simulink model "simTwoLinkFDIbasisComparison"  (R2014b)
settings: Solver=ode45  StartTime=0.0  StopTime=tof  FixedStep=dt  MaxStep=dtmax  RelTol=1e-3
values from neighbouring files (symbols this model uses):
  As = zeros(nofstates,nofstates)    [threeLinkFTC.m]    (also in twoLinkFDIbasisComparison.m; twoLinkFTC.m; twoLinkFTCwAdaptive.m)
  c1 = 0    [robotArmWith2Links.m]    (also in twoLinkFDIbasisComparison.m = 1; twoLinkFTC.m; twoLinkFTCwAdaptive.m)
  c2 = 0    [robotArmWith2Links.m]    (also in twoLinkFDIbasisComparison.m = 1; twoLinkFTC.m; twoLinkFTCwAdaptive.m)
  Dhat0 = zeros(6,1)    [threeLinkFTC.m]    (also in twoLinkFDIbasisComparison.m = zeros(4,1); twoLinkFTC.m = zeros(4,1); twoLinkFTCwAdaptive.m = zeros(4,1))
  dtFc = 1*dtmax    (= 0.001)    [threeLinkFTC.m]    (also in twoLinkFDIbasisComparison.m; twoLinkFTC.m; twoLinkFTCwAdaptive.m)
  epsilontheta = 0.01    [threeLinkFTC.m]    (also in twoLinkFDIbasisComparison.m; twoLinkFTC.m; twoLinkFTCwAdaptive.m)
  fault_gamma = 1    [twoLinkFDIbasisComparison.m]
  fault_taumax = 15    [twoLinkFDIbasisComparison.m]
  faultyArm = 3    [threeLinkFTC.m]    (also in twoLinkFDIbasisComparison.m = 2; twoLinkFTC.m = 2; twoLinkFTCwAdaptive.m = 1)
  g = 9.81    [robotArmWith2Links.m]    (also in threeLinkFTC.m; twoLinkFDIbasisComparison.m; twoLinkFTC.m; twoLinkFTCwAdaptive.m)
  GammaW = 1000    [threeLinkFTC.m]    (also in twoLinkFDIbasisComparison.m; twoLinkFTC.m; twoLinkFTCwAdaptive.m)
  I1 = 8.33e-2    (= 0.0833)    [robotArmWith2Links.m]    (also in threeLinkFTC.m = 0.0833333333333; twoLinkFDIbasisComparison.m = 0.0833333333333; twoLinkFTC.m = 0.0833333333333; twoLinkFTCwAdaptive.m = 0.0833333333333)
  I2 = 8.33e-2    (= 0.0833)    [robotArmWith2Links.m]    (also in threeLinkFTC.m = 0.0833333333333; twoLinkFDIbasisComparison.m = 0.0833333333333; twoLinkFTC.m = 0.0833333333333; twoLinkFTCwAdaptive.m = 0.0833333333333)
  ifault = 2    [threeLinkFTC.m]    (also in twoLinkFDIbasisComparison.m; twoLinkFTC.m; twoLinkFTCwAdaptive.m)
  Kp = wn^2    (= 157.913670417)    [threeLinkFTC.m]    (also in twoLinkFDIbasisComparison.m = 3947.84176044; twoLinkFTC.m = 3947.84176044; twoLinkFTCwAdaptive.m = 3947.84176044)
  Kv = 2*ksi*wn    (= 17.5929188601)    [threeLinkFTC.m]    (also in twoLinkFDIbasisComparison.m = 125.663706144; twoLinkFTC.m = 125.663706144; twoLinkFTCwAdaptive.m = 125.663706144)
  l1 = 1    [robotArmWith2Links.m]    (also in threeLinkFTC.m; twoLinkFDIbasisComparison.m; twoLinkFTC.m; twoLinkFTCwAdaptive.m)
  l2 = 1    [robotArmWith2Links.m]    (also in threeLinkFTC.m; twoLinkFDIbasisComparison.m; twoLinkFTC.m; twoLinkFTCwAdaptive.m)
  lc1 = l1/2    (= 0.5)    [robotArmWith2Links.m]    (also in threeLinkFTC.m; twoLinkFDIbasisComparison.m; twoLinkFTC.m; twoLinkFTCwAdaptive.m)
  lc2 = l2/2    (= 0.5)    [robotArmWith2Links.m]    (also in threeLinkFTC.m; twoLinkFDIbasisComparison.m; twoLinkFTC.m; twoLinkFTCwAdaptive.m)
  m1 = 1    [robotArmWith2Links.m]    (also in threeLinkFTC.m; twoLinkFDIbasisComparison.m; twoLinkFTC.m; twoLinkFTCwAdaptive.m)
  m2 = 1    [robotArmWith2Links.m]    (also in threeLinkFTC.m; twoLinkFDIbasisComparison.m; twoLinkFTC.m; twoLinkFTCwAdaptive.m)
  nCheby = 4    [threeLinkFTC.m]    (also in twoLinkFDIbasisComparison.m; twoLinkFTC.m; twoLinkFTCwAdaptive.m)
  nRBF = length(x1is)*length(x2is)*length(x3is)*length(x4is)    [twoLinkFDIbasisComparison.m]
  Ps = lyap(As(4:6,4:6)',Q)    [threeLinkFTC.m]    (also in twoLinkFDIbasisComparison.m = lyap(As(3:4,3:4)',Q); twoLinkFTC.m = lyap(As(3:4,3:4)',Q); twoLinkFTCwAdaptive.m = lyap(As(3:4,3:4)',Q))
  q0 = [80 20]'*pi/180    [robotArmWith2Links.m]    (also in threeLinkFTC.m = [90 0 0]'*pi/180; twoLinkFDIbasisComparison.m = [90 0]'*pi/180; twoLinkFTC.m = [90 0]'*pi/180; twoLinkFTCwAdaptive.m = [90 0]'*pi/180)
  qdot0 = [0 0]'    [robotArmWith2Links.m]    (also in threeLinkFTC.m = [0 0 0]'*pi/180; twoLinkFDIbasisComparison.m = [0 0]'*pi/180; twoLinkFTC.m = [0 0]'*pi/180; twoLinkFTCwAdaptive.m = [0 0]'*pi/180)
  tfault = 5    [threeLinkFTC.m]    (also in twoLinkFDIbasisComparison.m; twoLinkFTC.m; twoLinkFTCwAdaptive.m = 1)
  visualFlag = 0    [robotArmWith2Links.m]    (also in twoLinkFDIbasisComparison.m; twoLinkFTC.m; twoLinkFTCwAdaptive.m)
  visualizationDataFlag = 1    [robotArmWith2Links.m]    (also in twoLinkFDIbasisComparison.m; twoLinkFTC.m; twoLinkFTCwAdaptive.m)
  W0 = 0    [threeLinkFTC.m]    (also in twoLinkFDIbasisComparison.m; twoLinkFTC.m; twoLinkFTCwAdaptive.m)
  Wbnd = 1000    [threeLinkFTC.m]    (also in twoLinkFDIbasisComparison.m; twoLinkFTC.m; twoLinkFTCwAdaptive.m)
  xhat0 = [q0 ; qdot0]    [threeLinkFTC.m]    (also in twoLinkFDIbasisComparison.m; twoLinkFTC.m; twoLinkFTCwAdaptive.m)
  xu = zeros(nRBF,2)    [twoLinkFDIbasisComparison.m]
undefined symbols (not defined in the file or in its folder): Intmax, Intmin, twolinkplot
libraries: simulink x4, vrlib x4, dspbuff3 x2
(part 2 of 2)

== system simTwoLinkFDIbasisComparison/System/System Parameters/getH ==
  c2 : Inport
  m1 : Inport  Port=2
  m2 : Inport  Port=3
  I1 : Inport  Port=4
  I2 : Inport  Port=5
  Gain : Gain  Gain=2
  Gain1 : Gain  Gain=lc2^2
  Gain4 : Gain  Gain=l1*lc2
  Gain5 : Gain  Gain=lc1^2
  Gain6 : Gain  Gain=l1^2+lc2^2
  Gain7 : Gain  Gain=lc2^2
  Matrix Concatenate : Concatenate  Mode=Multidimensional array  ConcatenateDimension=2
  Matrix Concatenate1 : Concatenate  Mode=Multidimensional array  ConcatenateDimension=2
  Matrix Concatenate2 : Concatenate  Mode=Multidimensional array
  Product : Product  RndMeth=Zero
  Sum : Sum  Inputs=+++++
  Sum1 : Sum  Inputs=+++
  Sum2 : Sum
  H : Outport
  wires:
  [H11] -> Matrix Concatenate/1
  [H12] -> Matrix Concatenate/2
  Matrix Concatenate/1 -> Matrix Concatenate2/1
  Matrix Concatenate1/1 -> Matrix Concatenate2/2
  [H21] -> Matrix Concatenate1/1
  [H22] -> Matrix Concatenate1/2
  Matrix Concatenate2/1 -> H/1
  c2/1 -> [c2]
  Sum/1 -> [H11]
  Sum1/1 -> [H12], [H21]
  [m2] -> Gain4/1
  Gain4/1 -> Product/1
  [c2] -> Product/2
  Product/1 -> [a]
  [m1] -> Gain5/1
  [m2] -> Gain6/1
  [I1] -> Sum/1
  [I2] -> Sum/2
  Gain5/1 -> Sum/3
  [a] -> Gain/1
  Gain6/1 -> Sum/4
  Gain/1 -> Sum/5
  [m2] -> Gain7/1
  [I2] -> Sum1/1
  Gain7/1 -> Sum1/2
  [a] -> Sum1/3
  [m2] -> Gain1/1
  [I2] -> Sum2/1
  Gain1/1 -> Sum2/2
  Sum2/1 -> [H22]
  m1/1 -> [m1]
  m2/1 -> [m2]
  I1/1 -> [I1]
  I2/1 -> [I2]

== system simTwoLinkFDIbasisComparison/System/System Parameters/getH1 ==
  c2 : Inport
  m1 : Inport  Port=2
  m2 : Inport  Port=3
  I1 : Inport  Port=4
  I2 : Inport  Port=5
  Gain : Gain  Gain=2
  Gain1 : Gain  Gain=lc2^2
  Gain4 : Gain  Gain=l1*lc2
  Gain5 : Gain  Gain=lc1^2
  Gain6 : Gain  Gain=l1^2+lc2^2
  Gain7 : Gain  Gain=lc2^2
  Matrix Concatenate : Concatenate  Mode=Multidimensional array  ConcatenateDimension=2
  Matrix Concatenate1 : Concatenate  Mode=Multidimensional array  ConcatenateDimension=2
  Matrix Concatenate2 : Concatenate  Mode=Multidimensional array
  Product : Product  RndMeth=Zero
  Sum : Sum  Inputs=+++++
  Sum1 : Sum  Inputs=+++
  Sum2 : Sum
  H : Outport
  wires:
  [H11] -> Matrix Concatenate/1
  [H12] -> Matrix Concatenate/2
  Matrix Concatenate/1 -> Matrix Concatenate2/1
  Matrix Concatenate1/1 -> Matrix Concatenate2/2
  [H21] -> Matrix Concatenate1/1
  [H22] -> Matrix Concatenate1/2
  Matrix Concatenate2/1 -> H/1
  c2/1 -> [c2]
  Sum/1 -> [H11]
  Sum1/1 -> [H12], [H21]
  [m2] -> Gain4/1
  Gain4/1 -> Product/1
  [c2] -> Product/2
  Product/1 -> [a]
  [m1] -> Gain5/1
  [m2] -> Gain6/1
  [I1] -> Sum/1
  [I2] -> Sum/2
  Gain5/1 -> Sum/3
  [a] -> Gain/1
  Gain6/1 -> Sum/4
  Gain/1 -> Sum/5
  [m2] -> Gain7/1
  [I2] -> Sum1/1
  Gain7/1 -> Sum1/2
  [a] -> Sum1/3
  [m2] -> Gain1/1
  [I2] -> Sum2/1
  Gain1/1 -> Sum2/2
  Sum2/1 -> [H22]
  m1/1 -> [m1]
  m2/1 -> [m2]
  I1/1 -> [I1]
  I2/1 -> [I2]

== system simTwoLinkFDIbasisComparison/System/System Parameters/getMass ==
  Constant : Constant  Value=m1
  Constant1 : Constant  Value=m2
  Constant5 : Constant  Value=I1
  Constant6 : Constant  Value=I2
  m1 : Outport
  m2 : Outport  Port=2
  I1 : Outport  Port=3
  I2 : Outport  Port=4
  wires:
  [m1] -> m1/1  "m1"
  [m2] -> m2/1  "m2"
  [I1] -> I1/1  "I1"
  [I2] -> I2/1  "I2"
  Constant5/1 -> [I1]
  Constant/1 -> [m1]
  Constant1/1 -> [m2]
  Constant6/1 -> [I2]

== system simTwoLinkFDIbasisComparison/Controller/Disturbance Estimator/getDisturbance/Chebyshev Basis Functions ==
  x : Inport
  tau : Inport  Port=2
  Chebyshev Polynomail Value Calculation : Subsystem  TreatAsAtomicUnit=on
  Demux : Demux
  Mux : Mux
  Reshape1 : Reshape  OutputDimensionality=Column vector (2-D)
  Reshape2 : Reshape  OutputDimensionality=Column vector (2-D)
  Terminator1 : Terminator
  Tn : Outport
  wires:
  [Tn] -> Tn/1
  [z] -> Chebyshev Polynomail Value Calculation/1(x)
  Chebyshev Polynomail Value Calculation/1(chebyPol) -> Reshape2/1
  Reshape2/1 -> [Tn]
  tau/1 -> Terminator1/1
  x/1 -> [x]
  [x] -> Demux/1
  Demux/1 -> [q1]
  Demux/2 -> [q2]
  Demux/3 -> [q1dot]
  Demux/4 -> [q2dot]
  Mux/1 -> Reshape1/1
  Reshape1/1 -> [z]
  [q1] -> Mux/1
  [q2] -> Mux/2
  [q1dot] -> Mux/3
  [q2dot] -> Mux/4

== system simTwoLinkFDIbasisComparison/Controller/Disturbance Estimator/getDisturbance/Custom Basis Functions ==
  x : Inport
  tau : Inport  Port=2
  Add : Sum
  Constant : Constant
  Demux : Demux
  Math Function : Math  Operator=square  SaturateOnIntegerOverflow=on
  Math Function1 : Math  Operator=square  SaturateOnIntegerOverflow=on
  Mux : Mux  Inputs=7
  Product{1..4} (4 alike) : Product  RndMeth=Zero
  Reshape : Reshape  OutputDimensionality=Column vector (2-D)
  Terminator1 : Terminator
  Trigonometric Function : Trigonometry  Operator=cos
  Trigonometric Function1 : Trigonometry  Operator=cos
  Trigonometric Function{2..5} (4 alike) : Trigonometry
  psiz : Outport
  wires:
  [psiz] -> psiz/1
  Constant/1 -> Mux/1
  Mux/1 -> Reshape/1
  Reshape/1 -> [psiz]
  tau/1 -> Terminator1/1
  x/1 -> [x]
  [x] -> Demux/1
  Demux/1 -> [q1]
  Demux/2 -> [q2]
  Demux/3 -> [q1dot]
  Demux/4 -> [q2dot]
  [q1] -> Trigonometric Function/1
  Trigonometric Function/1 -> Mux/2
  [q1] -> Add/1
  [q2] -> Add/2
  Add/1 -> Trigonometric Function1/1
  Trigonometric Function1/1 -> Mux/3
  [q2] -> Trigonometric Function2/1
  Trigonometric Function2/1 -> Product1/1
  [q1dot] -> Product1/2
  Product1/1 -> Mux/4
  [q2] -> Trigonometric Function3/1
  Trigonometric Function3/1 -> Product2/1
  [q2dot] -> Product2/2
  Product2/1 -> Mux/5
  [q2] -> Trigonometric Function4/1
  Trigonometric Function4/1 -> Product3/1
  [q1dot] -> Math Function/1
  Math Function/1 -> Product3/2
  Product3/1 -> Mux/6
  [q2] -> Trigonometric Function5/1
  Trigonometric Function5/1 -> Product4/1
  [q2dot] -> Math Function1/1
  Math Function1/1 -> Product4/2
  Product4/1 -> Mux/7

== system simTwoLinkFDIbasisComparison/Controller/Disturbance Estimator/getDisturbance/RBF Basis Functions ==
  x : Inport
  tau : Inport  Port=2
  Demux : Demux
  Mux : Mux
  RBF Calculation : Subsystem  TreatAsAtomicUnit=on
  Reshape1 : Reshape  OutputDimensionality=Column vector (2-D)
  Reshape2 : Reshape  OutputDimensionality=Column vector (2-D)
  Terminator1 : Terminator
  phiz : Outport
  wires:
  [phiz] -> phiz/1
  [z] -> RBF Calculation/1(z)
  RBF Calculation/1(RBFs) -> Reshape2/1
  Reshape2/1 -> [phiz]
  tau/1 -> Terminator1/1
  x/1 -> [x]
  [x] -> Demux/1
  Demux/1 -> [q1]
  Demux/2 -> [q2]
  Demux/3 -> [q1dot]
  Demux/4 -> [q2dot]
  Mux/1 -> Reshape1/1
  Reshape1/1 -> [z]
  [q1] -> Mux/1
  [q2] -> Mux/2
  [q1dot] -> Mux/3
  [q2dot] -> Mux/4

== system simTwoLinkFDIbasisComparison/Controller/Disturbance Estimator/getDisturbance/getDhat ==
  psiz : Inport
  es : Inport  Port=2
  Math Function : Math  Operator=transpose  SaturateOnIntegerOverflow=on
  Math Function1 : Math  Operator=transpose  SaturateOnIntegerOverflow=on
  Reshape : Reshape  OutputDimensionality=Column vector (2-D)
  Selector : Selector  NumberOfDimensions=2  InputPortWidth=3  IndexOptions=Select all,Index vector (dialog)  Indices=[1 3],1  OutputSizes=1,1
  Selector1 : Selector  NumberOfDimensions=2  InputPortWidth=3  IndexOptions=Select all,Index vector (dialog)  Indices=[1 3],2  OutputSizes=1,1
  Terminator1 : Terminator
  Vector Concatenate : Concatenate
  Vector Concatenate1 : Concatenate  Mode=Multidimensional array
  adaptiveGain : Subsystem  TreatAsAtomicUnit=on
  getW1 : Subsystem
  getW2 : Subsystem
  Dhat : Outport
  wires:
  es/1 -> [es]  "es"
  adaptiveGain/1(Wintegrand) -> [Wint]  "Wint"
  [Dhat] -> Dhat/1  "Dhat"
  psiz/1 -> [psiz]  "psiz"
  [es] -> adaptiveGain/2(es)
  [psiz] -> adaptiveGain/1(psi(z))
  [psiz] -> getW1/2(psiz)
  Selector/1 -> getW1/1(Wint)
  Vector Concatenate/1 -> Reshape/1
  [psiz] -> getW2/2(psiz)
  Selector1/1 -> getW2/1(Wint)
  Reshape/1 -> [Dhat]
  Vector Concatenate1/1 -> Terminator1/1  "W"
  getW2/2(WTpsi) -> Vector Concatenate/2
  getW1/2(WTpsi) -> Vector Concatenate/1
  getW1/1(W) -> Math Function/1
  getW2/1(W) -> Math Function1/1
  [Wint] -> Selector1/1, Selector/1
  Math Function/1 -> Vector Concatenate1/1
  Math Function1/1 -> Vector Concatenate1/2

== system simTwoLinkFDIbasisComparison/Controller/Disturbance Estimator/getDisturbance/getDhat1 ==
  psiz : Inport
  es : Inport  Port=2
  Math Function : Math  Operator=transpose  SaturateOnIntegerOverflow=on
  Math Function1 : Math  Operator=transpose  SaturateOnIntegerOverflow=on
  Reshape : Reshape  OutputDimensionality=Column vector (2-D)
  Selector : Selector  NumberOfDimensions=2  InputPortWidth=3  IndexOptions=Select all,Index vector (dialog)  Indices=[1 3],1  OutputSizes=1,1
  Selector1 : Selector  NumberOfDimensions=2  InputPortWidth=3  IndexOptions=Select all,Index vector (dialog)  Indices=[1 3],2  OutputSizes=1,1
  Terminator1 : Terminator
  Vector Concatenate : Concatenate
  Vector Concatenate1 : Concatenate  Mode=Multidimensional array
  adaptiveGain : Subsystem  TreatAsAtomicUnit=on
  getW1 : Subsystem
  getW2 : Subsystem
  Dhat : Outport
  wires:
  es/1 -> [es]  "es"
  adaptiveGain/1(Wintegrand) -> [Wint]  "Wint"
  [Dhat] -> Dhat/1  "Dhat"
  psiz/1 -> [psiz]  "psiz"
  [es] -> adaptiveGain/2(es)
  [psiz] -> adaptiveGain/1(psi(z))
  [psiz] -> getW1/2(psiz)
  Selector/1 -> getW1/1(Wint)
  Vector Concatenate/1 -> Reshape/1
  [psiz] -> getW2/2(psiz)
  Selector1/1 -> getW2/1(Wint)
  Reshape/1 -> [Dhat]
  Vector Concatenate1/1 -> Terminator1/1  "W"
  getW2/2(WTpsi) -> Vector Concatenate/2
  getW1/2(WTpsi) -> Vector Concatenate/1
  getW1/1(W) -> Math Function/1
  getW2/1(W) -> Math Function1/1
  [Wint] -> Selector1/1, Selector/1
  Math Function/1 -> Vector Concatenate1/1
  Math Function1/1 -> Vector Concatenate1/2

== system simTwoLinkFDIbasisComparison/Controller/Disturbance Estimator/getDisturbance/Chebyshev Basis Functions/Chebyshev Polynomail Value Calculation ==
  x : Inport
  Delay Line : dspbuff3/Delay Line  siz=nCheby  ic=zeros(nCheby,1)  directfeed=on  enable_output=off  hold_output=off  TreatMby1Signals=M channels (this choice will be removed - see release notes)
  For Iterator : ForIterator  IterationLimit=nCheby
  Frame Conversion : FrameConversion  OutFrame=Sample-based
  If : If  IfExpression=u1 > 2
  If Action Subsystem : Subsystem  TreatAsAtomicUnit=on
  If Action Subsystem1 : Subsystem  TreatAsAtomicUnit=on
  Memory : Memory  InheritSampleTime=on  LinearizeMemory=on  LinearizeAsDelay=on
  Merge : Merge
  Reshape : Reshape  OutputDimensionality=Column vector (2-D)
  chebyPol : Outport
  wires:
  For Iterator/1 -> [N]
  x/1 -> [x]
  [N] -> If/1
  If/1 -> If Action Subsystem/Action
  If/2 -> If Action Subsystem1/Action
  [N] -> If Action Subsystem1/2(N)
  [x] -> If Action Subsystem1/1(x)
  [x] -> If Action Subsystem/1(x)
  If Action Subsystem/1(polyval) -> Merge/1
  If Action Subsystem1/1(polval) -> Merge/2
  Merge/1 -> [polyval]
  [polyval] -> Delay Line/1
  Delay Line/1 -> Frame Conversion/1
  Reshape/1 -> [polyvals]
  [polyvals] -> Memory/1
  [polyvals] -> chebyPol/1  "chebyPol"
  Frame Conversion/1 -> Reshape/1
  Memory/1 -> If Action Subsystem/2(polyvals)

== system simTwoLinkFDIbasisComparison/Controller/Disturbance Estimator/getDisturbance/RBF Basis Functions/RBF Calculation ==
  z : Inport
  Add{,1,3..4} (4 alike) : Sum  Inputs=+-
  Add2 : Sum  Inputs=++++
  Constant : Constant  Value=xu  VectorParams1D=off
  Delay Line : dspbuff3/Delay Line  siz=nRBF  ic=zeros(nRBF,1)  directfeed=on  enable_output=off  hold_output=off  TreatMby1Signals=M channels (this choice will be removed - see release notes)
  Demux : Demux
  Demux1 : Demux
  For Iterator : ForIterator  IterationLimit=nRBF
  Frame Conversion : FrameConversion  OutFrame=Sample-based
  Gain : Gain  Gain=-3/2
  Math Function{,1,3..4} (4 alike) : Math  Operator=square  SaturateOnIntegerOverflow=on
  Math Function2 : Math  SaturateOnIntegerOverflow=on
  Reshape : Reshape  OutputDimensionality=Column vector (2-D)
  Selector : Selector  NumberOfDimensions=2  IndexOptions=Index vector (port),Select all  Indices=[1 3],1  OutputSizes=1,1
  RBFs : Outport
  wires:
  For Iterator/1 -> [N]
  [RBF] -> Delay Line/1
  Delay Line/1 -> Frame Conversion/1
  Frame Conversion/1 -> Reshape/1
  [xu] -> Selector/1  "xu"
  [N] -> Selector/2  "N"
  [x1] -> Add/1
  [x1i] -> Add/2
  Add/1 -> Math Function/1
  [x2] -> Add1/1
  [x2i] -> Add1/2
  Add1/1 -> Math Function1/1
  Math Function/1 -> Add2/1
  Math Function1/1 -> Add2/2
  Add2/1 -> Gain/1
  Gain/1 -> Math Function2/1
  Math Function2/1 -> [RBF]
  Reshape/1 -> RBFs/1  "RBFs"
  Constant/1 -> [xu]
  Selector/1 -> Demux/1  "xis"
  Demux/1 -> [x1i]
  Demux/2 -> [x2i]
  [z] -> Demux1/1
  Demux1/1 -> [x1]
  Demux1/2 -> [x2]
  Demux1/3 -> [x3]
  Demux1/4 -> [x4]
  [x3] -> Add3/1
  [x3i] -> Add3/2
  Add3/1 -> Math Function3/1
  [x4] -> Add4/1
  [x4i] -> Add4/2
  Add4/1 -> Math Function4/1
  Math Function3/1 -> Add2/3
  Math Function4/1 -> Add2/4
  Demux/3 -> [x3i]
  Demux/4 -> [x4i]
  z/1 -> [z]

== system simTwoLinkFDIbasisComparison/Controller/Disturbance Estimator/getDisturbance/getDhat/adaptiveGain ==
  psi(z) : Inport
  es : Inport  Port=2
  Gain1 : Gain  Gain=-1
  Math Function : Math  Operator=transpose  SaturateOnIntegerOverflow=on
  P : Constant  Value=Ps  VectorParams1D=off
  Product1 : Product  Multiplication=Matrix(*)  RndMeth=Zero
  Product3 : Product  Multiplication=Matrix(*)  RndMeth=Zero
  Wintegrand : Outport
  wires:
  Product1/1 -> Product3/2
  psi(z)/1 -> Product3/1
  Gain1/1 -> Wintegrand/1
  es/1 -> Math Function/1
  Math Function/1 -> Product1/1
  P/1 -> Product1/2
  Product3/1 -> Gain1/1

== system simTwoLinkFDIbasisComparison/Controller/Disturbance Estimator/getDisturbance/getDhat/getW1 ==
  Wint : Inport
  psiz : Inport  Port=2
  Constant : Constant  Value=Wbnd  VectorParams1D=off
  Constant1 : Constant  Value=epsilontheta
  Discrete-Time Integrator : DiscreteIntegrator  IntegratorMethod=Integration: Trapezoidal  InitialCondition=W0  SampleTime=-1  LimitOutput=on  UpperSaturationLimit=Wbnd  LowerSaturationLimit=-Wbnd
  Gain : Gain  Gain=GammaW
  Math Function : Math  Operator=transpose  SaturateOnIntegerOverflow=on
  Memory4 : Memory  X0=W0  InheritSampleTime=on  LinearizeMemory=on  LinearizeAsDelay=on
  Product : Product  Multiplication=Matrix(*)  RndMeth=Zero
  Projection : Subsystem  TreatAsAtomicUnit=on
  W : Outport
  WTpsi : Outport  Port=2
  wires:
  [WTpsi] -> WTpsi/1
  [Wint] -> Projection/2(y)
  Math Function/1 -> Product/1
  [psiz] -> Product/2
  Discrete-Time Integrator/1 -> Math Function/1, [W], Memory4/1
  Gain/1 -> Discrete-Time Integrator/1
  Projection/1(Proj) -> Gain/1  "WintProj"
  Memory4/1 -> Projection/1(theta)
  Constant/1 -> Projection/3(Thetamax)
  Constant1/1 -> Projection/4(epsilontheta)
  [W] -> W/1
  Wint/1 -> [Wint]
  psiz/1 -> [psiz]
  Product/1 -> [WTpsi]  "WTpsi"

== system simTwoLinkFDIbasisComparison/Controller/Disturbance Estimator/getDisturbance/getDhat/getW2 ==
  Wint : Inport
  psiz : Inport  Port=2
  Constant : Constant  Value=Wbnd  VectorParams1D=off
  Constant1 : Constant  Value=epsilontheta
  Discrete-Time Integrator : DiscreteIntegrator  IntegratorMethod=Integration: Trapezoidal  InitialCondition=W0  SampleTime=-1  LimitOutput=on  UpperSaturationLimit=Wbnd  LowerSaturationLimit=-Wbnd
  Gain : Gain  Gain=GammaW
  Math Function : Math  Operator=transpose  SaturateOnIntegerOverflow=on
  Memory4 : Memory  X0=W0  InheritSampleTime=on  LinearizeMemory=on  LinearizeAsDelay=on
  Product : Product  Multiplication=Matrix(*)  RndMeth=Zero
  Projection : Subsystem  TreatAsAtomicUnit=on
  W : Outport
  WTpsi : Outport  Port=2
  wires:
  Product/1 -> [WTpsi]  "WTpsi"
  psiz/1 -> [psiz]
  Wint/1 -> [Wint]
  [W] -> W/1
  Constant1/1 -> Projection/4(epsilontheta)
  Constant/1 -> Projection/3(Thetamax)
  Memory4/1 -> Projection/1(theta)
  Projection/1(Proj) -> Gain/1  "WintProj"
  Gain/1 -> Discrete-Time Integrator/1
  Discrete-Time Integrator/1 -> Memory4/1, [W], Math Function/1
  [psiz] -> Product/2
  Math Function/1 -> Product/1
  [Wint] -> Projection/2(y)
  [WTpsi] -> WTpsi/1

== system simTwoLinkFDIbasisComparison/Controller/Disturbance Estimator/getDisturbance/getDhat1/adaptiveGain ==
  psi(z) : Inport
  es : Inport  Port=2
  Gain1 : Gain  Gain=-1
  Math Function : Math  Operator=transpose  SaturateOnIntegerOverflow=on
  P : Constant  Value=Ps  VectorParams1D=off
  Product1 : Product  Multiplication=Matrix(*)  RndMeth=Zero
  Product3 : Product  Multiplication=Matrix(*)  RndMeth=Zero
  Wintegrand : Outport
  wires:
  Product1/1 -> Product3/2
  psi(z)/1 -> Product3/1
  Gain1/1 -> Wintegrand/1
  es/1 -> Math Function/1
  Math Function/1 -> Product1/1
  P/1 -> Product1/2
  Product3/1 -> Gain1/1

== system simTwoLinkFDIbasisComparison/Controller/Disturbance Estimator/getDisturbance/getDhat1/getW1 ==
  Wint : Inport
  psiz : Inport  Port=2
  Constant : Constant  Value=Wbnd  VectorParams1D=off
  Constant1 : Constant  Value=epsilontheta
  Discrete-Time Integrator : DiscreteIntegrator  IntegratorMethod=Integration: Trapezoidal  InitialCondition=W0  SampleTime=-1  LimitOutput=on  UpperSaturationLimit=Wbnd  LowerSaturationLimit=-Wbnd
  Gain : Gain  Gain=GammaW
  Math Function : Math  Operator=transpose  SaturateOnIntegerOverflow=on
  Memory4 : Memory  X0=W0  InheritSampleTime=on  LinearizeMemory=on  LinearizeAsDelay=on
  Product : Product  Multiplication=Matrix(*)  RndMeth=Zero
  Projection : Subsystem  TreatAsAtomicUnit=on
  W : Outport
  WTpsi : Outport  Port=2
  wires:
  [WTpsi] -> WTpsi/1
  [Wint] -> Projection/2(y)
  Math Function/1 -> Product/1
  [psiz] -> Product/2
  Discrete-Time Integrator/1 -> Math Function/1, [W], Memory4/1
  Gain/1 -> Discrete-Time Integrator/1
  Projection/1(Proj) -> Gain/1  "WintProj"
  Memory4/1 -> Projection/1(theta)
  Constant/1 -> Projection/3(Thetamax)
  Constant1/1 -> Projection/4(epsilontheta)
  [W] -> W/1
  Wint/1 -> [Wint]
  psiz/1 -> [psiz]
  Product/1 -> [WTpsi]  "WTpsi"

== system simTwoLinkFDIbasisComparison/Controller/Disturbance Estimator/getDisturbance/getDhat1/getW2 ==
  Wint : Inport
  psiz : Inport  Port=2
  Constant : Constant  Value=Wbnd  VectorParams1D=off
  Constant1 : Constant  Value=epsilontheta
  Discrete-Time Integrator : DiscreteIntegrator  IntegratorMethod=Integration: Trapezoidal  InitialCondition=W0  SampleTime=-1  LimitOutput=on  UpperSaturationLimit=Wbnd  LowerSaturationLimit=-Wbnd
  Gain : Gain  Gain=GammaW
  Math Function : Math  Operator=transpose  SaturateOnIntegerOverflow=on
  Memory4 : Memory  X0=W0  InheritSampleTime=on  LinearizeMemory=on  LinearizeAsDelay=on
  Product : Product  Multiplication=Matrix(*)  RndMeth=Zero
  Projection : Subsystem  TreatAsAtomicUnit=on
  W : Outport
  WTpsi : Outport  Port=2
  wires:
  Product/1 -> [WTpsi]  "WTpsi"
  psiz/1 -> [psiz]
  Wint/1 -> [Wint]
  [W] -> W/1
  Constant1/1 -> Projection/4(epsilontheta)
  Constant/1 -> Projection/3(Thetamax)
  Memory4/1 -> Projection/1(theta)
  Projection/1(Proj) -> Gain/1  "WintProj"
  Gain/1 -> Discrete-Time Integrator/1
  Discrete-Time Integrator/1 -> Memory4/1, [W], Math Function/1
  [psiz] -> Product/2
  Math Function/1 -> Product/1
  [Wint] -> Projection/2(y)
  [WTpsi] -> WTpsi/1

== system simTwoLinkFDIbasisComparison/Controller/Disturbance Estimator/getDisturbance/Chebyshev Basis Functions/Chebyshev Polynomail Value Calculation/If Action Subsystem ==
  x : Inport
  polyvals : Inport  Port=2
  Action Port : ActionPort  PropagateVarSize=During execution  ActionType=then
  Add : Sum  Inputs=+-
  Constant : Constant  Value=nCheby
  Constant1 : Constant  Value=nCheby-1
  Gain : Gain  Gain=2
  Product : Product  RndMeth=Zero
  Selector : Selector  IndexOptions=Index vector (port)  Indices=[1 3]
  Selector1 : Selector  IndexOptions=Index vector (port)  Indices=[1 3]
  polyval : Outport
  wires:
  x/1 -> [x]
  polyvals/1 -> [polyvals]  "if.polyvals"
  [polyvals] -> Selector/1
  Constant1/1 -> Selector/2
  Selector/1 -> [Tm2]  "Tm2"
  [polyvals] -> Selector1/1
  Constant/1 -> Selector1/2
  Selector1/1 -> [Tm1]  "Tm1"
  [x] -> Product/1
  [Tm1] -> Product/2
  Product/1 -> Gain/1
  Gain/1 -> Add/1
  [Tm2] -> Add/2
  Add/1 -> polyval/1  "if.polyval"

== system simTwoLinkFDIbasisComparison/Controller/Disturbance Estimator/getDisturbance/Chebyshev Basis Functions/Chebyshev Polynomail Value Calculation/If Action Subsystem1 ==
  x : Inport
  N : Inport  Port=2
  Action Port : ActionPort  PropagateVarSize=During execution  ActionType=else
  Bias1 : Bias  Bias=-1
  Data Type Conversion : DataTypeConversion
  Math Function : Math  Operator=pow  OutputSignalType=real  SaturateOnIntegerOverflow=on
  polval : Outport
  wires:
  x/1 -> Math Function/1
  N/1 -> Bias1/1  "else.N"
  Math Function/1 -> polval/1  "else.polyval"
  Data Type Conversion/1 -> Math Function/2
  Bias1/1 -> Data Type Conversion/1

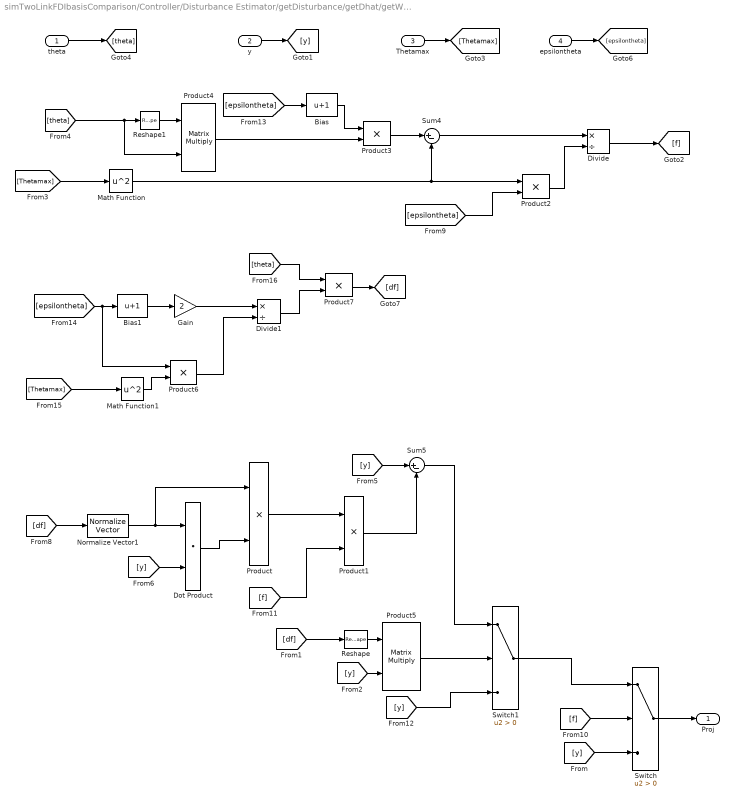
== system simTwoLinkFDIbasisComparison/Controller/Disturbance Estimator/getDisturbance/getDhat/getW1/Projection ==
  theta : Inport
  y : Inport  Port=2
  Thetamax : Inport  Port=3
  epsilontheta : Inport  Port=4
  Bias : Bias  Bias=1
  Bias1 : Bias  Bias=1
  Divide : Product  Inputs=*/
  Divide1 : Product  Inputs=*/
  Dot Product : DotProduct  InputSameDT=on  OutDataTypeStr=Inherit: Inherit via internal rule
  Gain : Gain  Gain=2
  Math Function : Math  Operator=square  SaturateOnIntegerOverflow=on
  Math Function1 : Math  Operator=square  SaturateOnIntegerOverflow=on
  Normalize Vector1 : vrlib/Utilities/Normalize Vector  maxzero=0
  Product{,1..3,6..7} (6 alike) : Product  RndMeth=Zero
  Product4 : Product  Multiplication=Matrix(*)  RndMeth=Zero
  Product5 : Product  Multiplication=Matrix(*)  RndMeth=Zero
  Reshape : Reshape  OutputDimensionality=Row vector (2-D)
  Reshape1 : Reshape  OutputDimensionality=Row vector (2-D)
  Sum4 : Sum  Inputs=|+-
  Sum5 : Sum  Inputs=|+-
  Switch : Switch  Criteria=u2 > Threshold
  Switch1 : Switch  Criteria=u2 > Threshold
  Proj : Outport
  wires:
  [f] -> Switch/2
  y/1 -> [y]
  Switch/1 -> Proj/1
  Product5/1 -> Switch1/2
  [y] -> Product5/2
  Sum4/1 -> Divide/1
  Math Function/1 -> Sum4/2, Product2/1
  Product4/1 -> Product3/2
  [theta] -> Reshape1/1, Product4/2
  [df] -> Reshape/1
  Reshape/1 -> Product5/1
  Reshape1/1 -> Product4/1
  theta/1 -> [theta]
  [y] -> Switch/3
  Switch1/1 -> Switch/1
  [y] -> Sum5/1
  Product/1 -> Product1/1
  [y] -> Switch1/3
  Product1/1 -> Sum5/2
  Sum5/1 -> Switch1/1
  [f] -> Product1/2
  [df] -> Normalize Vector1/1
  Normalize Vector1/1 -> Dot Product/1, Product/1
  [y] -> Dot Product/2
  Dot Product/1 -> Product/2
  Thetamax/1 -> [Thetamax]
  [Thetamax] -> Math Function/1
  epsilontheta/1 -> [epsilontheta]
  [epsilontheta] -> Product2/2
  Product2/1 -> Divide/2
  Divide/1 -> [f]
  Product3/1 -> Sum4/1
  Bias/1 -> Product3/1
  [epsilontheta] -> Bias/1
  [epsilontheta] -> Bias1/1, Product6/1
  Bias1/1 -> Gain/1
  Gain/1 -> Divide1/1
  [Thetamax] -> Math Function1/1
  Math Function1/1 -> Product6/2
  Product6/1 -> Divide1/2
  Product7/1 -> [df]
  [theta] -> Product7/1
  Divide1/1 -> Product7/2

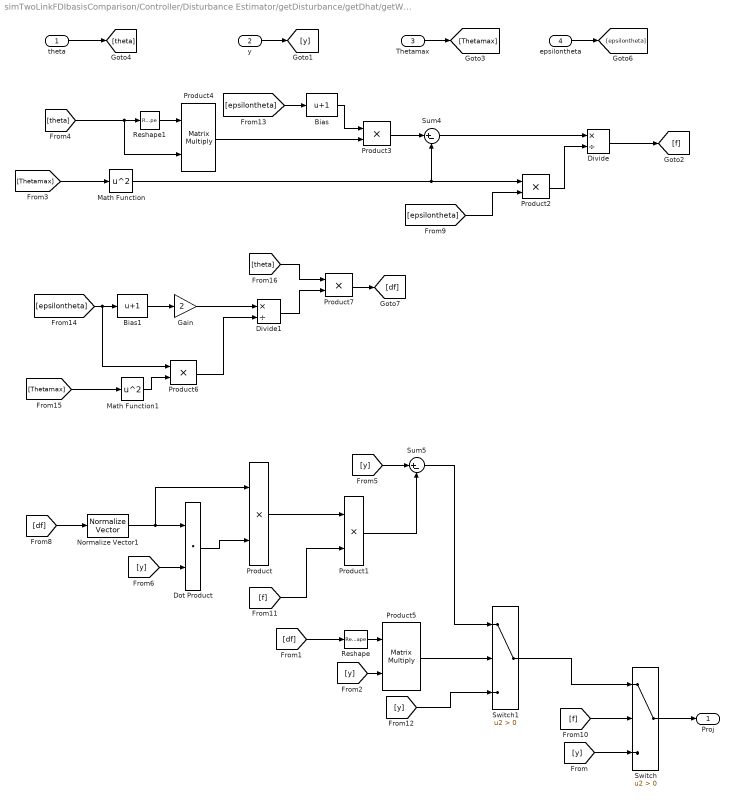
== system simTwoLinkFDIbasisComparison/Controller/Disturbance Estimator/getDisturbance/getDhat/getW2/Projection ==
  theta : Inport
  y : Inport  Port=2
  Thetamax : Inport  Port=3
  epsilontheta : Inport  Port=4
  Bias : Bias  Bias=1
  Bias1 : Bias  Bias=1
  Divide : Product  Inputs=*/
  Divide1 : Product  Inputs=*/
  Dot Product : DotProduct  InputSameDT=on  OutDataTypeStr=Inherit: Inherit via internal rule
  Gain : Gain  Gain=2
  Math Function : Math  Operator=square  SaturateOnIntegerOverflow=on
  Math Function1 : Math  Operator=square  SaturateOnIntegerOverflow=on
  Normalize Vector1 : vrlib/Utilities/Normalize Vector  maxzero=0
  Product{,1..3,6..7} (6 alike) : Product  RndMeth=Zero
  Product4 : Product  Multiplication=Matrix(*)  RndMeth=Zero
  Product5 : Product  Multiplication=Matrix(*)  RndMeth=Zero
  Reshape : Reshape  OutputDimensionality=Row vector (2-D)
  Reshape1 : Reshape  OutputDimensionality=Row vector (2-D)
  Sum4 : Sum  Inputs=|+-
  Sum5 : Sum  Inputs=|+-
  Switch : Switch  Criteria=u2 > Threshold
  Switch1 : Switch  Criteria=u2 > Threshold
  Proj : Outport
  wires:
  Divide1/1 -> Product7/2
  [theta] -> Product7/1
  Product7/1 -> [df]
  Product6/1 -> Divide1/2
  Math Function1/1 -> Product6/2
  [Thetamax] -> Math Function1/1
  Gain/1 -> Divide1/1
  Bias1/1 -> Gain/1
  [epsilontheta] -> Product6/1, Bias1/1
  [epsilontheta] -> Bias/1
  Bias/1 -> Product3/1
  Product3/1 -> Sum4/1
  Divide/1 -> [f]
  Product2/1 -> Divide/2
  [epsilontheta] -> Product2/2
  epsilontheta/1 -> [epsilontheta]
  [Thetamax] -> Math Function/1
  Thetamax/1 -> [Thetamax]
  Dot Product/1 -> Product/2
  [y] -> Dot Product/2
  Normalize Vector1/1 -> Product/1, Dot Product/1
  [df] -> Normalize Vector1/1
  [f] -> Product1/2
  Sum5/1 -> Switch1/1
  Product1/1 -> Sum5/2
  [y] -> Switch1/3
  Product/1 -> Product1/1
  [y] -> Sum5/1
  Switch1/1 -> Switch/1
  [y] -> Switch/3
  theta/1 -> [theta]
  Reshape1/1 -> Product4/1
  Reshape/1 -> Product5/1
  [df] -> Reshape/1
  [theta] -> Product4/2, Reshape1/1
  Product4/1 -> Product3/2
  Math Function/1 -> Product2/1, Sum4/2
  Sum4/1 -> Divide/1
  [y] -> Product5/2
  Product5/1 -> Switch1/2
  Switch/1 -> Proj/1
  y/1 -> [y]
  [f] -> Switch/2

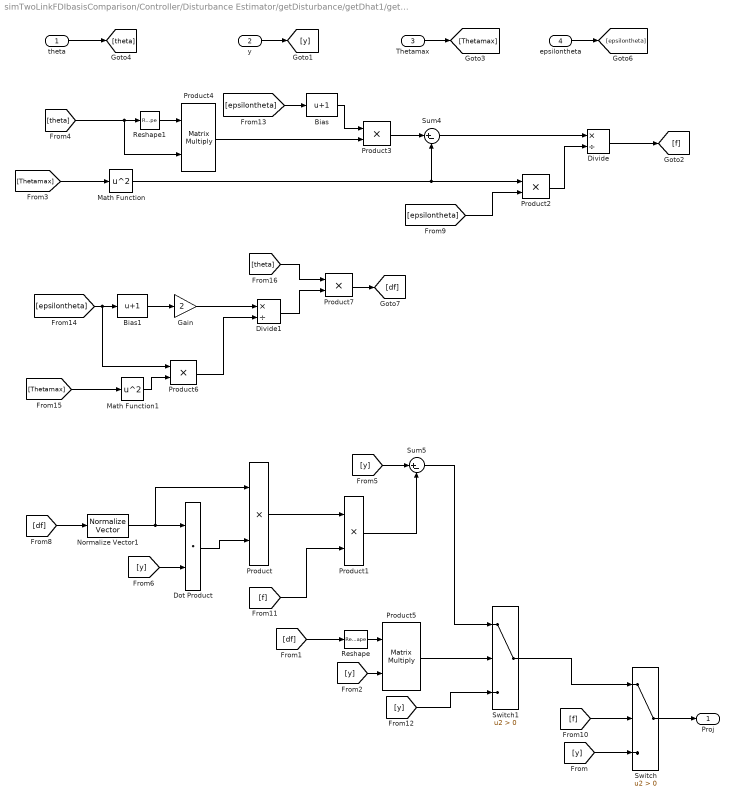
== system simTwoLinkFDIbasisComparison/Controller/Disturbance Estimator/getDisturbance/getDhat1/getW1/Projection ==
  theta : Inport
  y : Inport  Port=2
  Thetamax : Inport  Port=3
  epsilontheta : Inport  Port=4
  Bias : Bias  Bias=1
  Bias1 : Bias  Bias=1
  Divide : Product  Inputs=*/
  Divide1 : Product  Inputs=*/
  Dot Product : DotProduct  InputSameDT=on  OutDataTypeStr=Inherit: Inherit via internal rule
  Gain : Gain  Gain=2
  Math Function : Math  Operator=square  SaturateOnIntegerOverflow=on
  Math Function1 : Math  Operator=square  SaturateOnIntegerOverflow=on
  Normalize Vector1 : vrlib/Utilities/Normalize Vector  maxzero=0
  Product{,1..3,6..7} (6 alike) : Product  RndMeth=Zero
  Product4 : Product  Multiplication=Matrix(*)  RndMeth=Zero
  Product5 : Product  Multiplication=Matrix(*)  RndMeth=Zero
  Reshape : Reshape  OutputDimensionality=Row vector (2-D)
  Reshape1 : Reshape  OutputDimensionality=Row vector (2-D)
  Sum4 : Sum  Inputs=|+-
  Sum5 : Sum  Inputs=|+-
  Switch : Switch  Criteria=u2 > Threshold
  Switch1 : Switch  Criteria=u2 > Threshold
  Proj : Outport
  wires:
  [f] -> Switch/2
  y/1 -> [y]
  Switch/1 -> Proj/1
  Product5/1 -> Switch1/2
  [y] -> Product5/2
  Sum4/1 -> Divide/1
  Math Function/1 -> Sum4/2, Product2/1
  Product4/1 -> Product3/2
  [theta] -> Reshape1/1, Product4/2
  [df] -> Reshape/1
  Reshape/1 -> Product5/1
  Reshape1/1 -> Product4/1
  theta/1 -> [theta]
  [y] -> Switch/3
  Switch1/1 -> Switch/1
  [y] -> Sum5/1
  Product/1 -> Product1/1
  [y] -> Switch1/3
  Product1/1 -> Sum5/2
  Sum5/1 -> Switch1/1
  [f] -> Product1/2
  [df] -> Normalize Vector1/1
  Normalize Vector1/1 -> Dot Product/1, Product/1
  [y] -> Dot Product/2
  Dot Product/1 -> Product/2
  Thetamax/1 -> [Thetamax]
  [Thetamax] -> Math Function/1
  epsilontheta/1 -> [epsilontheta]
  [epsilontheta] -> Product2/2
  Product2/1 -> Divide/2
  Divide/1 -> [f]
  Product3/1 -> Sum4/1
  Bias/1 -> Product3/1
  [epsilontheta] -> Bias/1
  [epsilontheta] -> Bias1/1, Product6/1
  Bias1/1 -> Gain/1
  Gain/1 -> Divide1/1
  [Thetamax] -> Math Function1/1
  Math Function1/1 -> Product6/2
  Product6/1 -> Divide1/2
  Product7/1 -> [df]
  [theta] -> Product7/1
  Divide1/1 -> Product7/2

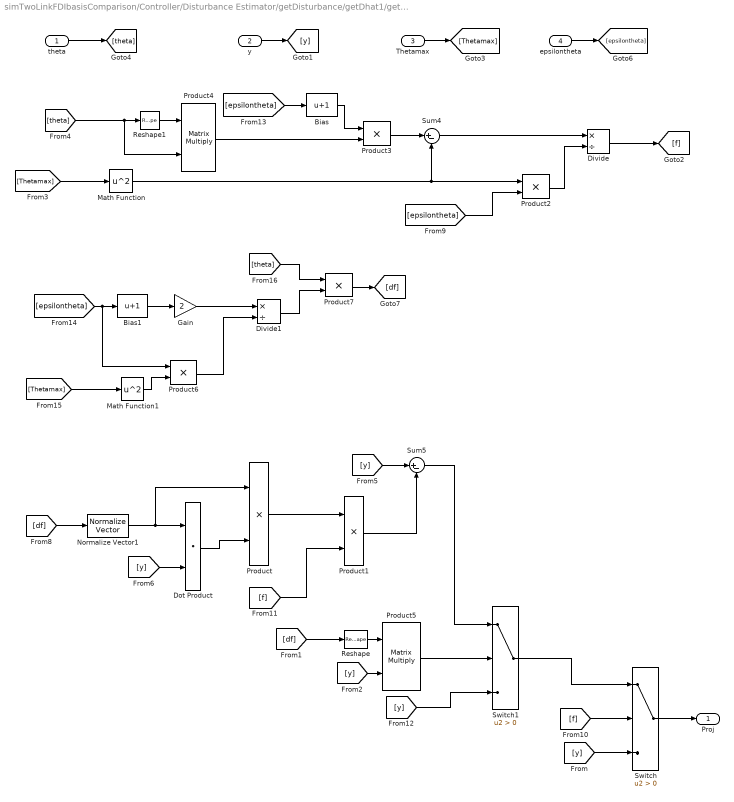
== system simTwoLinkFDIbasisComparison/Controller/Disturbance Estimator/getDisturbance/getDhat1/getW2/Projection ==
  theta : Inport
  y : Inport  Port=2
  Thetamax : Inport  Port=3
  epsilontheta : Inport  Port=4
  Bias : Bias  Bias=1
  Bias1 : Bias  Bias=1
  Divide : Product  Inputs=*/
  Divide1 : Product  Inputs=*/
  Dot Product : DotProduct  InputSameDT=on  OutDataTypeStr=Inherit: Inherit via internal rule
  Gain : Gain  Gain=2
  Math Function : Math  Operator=square  SaturateOnIntegerOverflow=on
  Math Function1 : Math  Operator=square  SaturateOnIntegerOverflow=on
  Normalize Vector1 : vrlib/Utilities/Normalize Vector  maxzero=0
  Product{,1..3,6..7} (6 alike) : Product  RndMeth=Zero
  Product4 : Product  Multiplication=Matrix(*)  RndMeth=Zero
  Product5 : Product  Multiplication=Matrix(*)  RndMeth=Zero
  Reshape : Reshape  OutputDimensionality=Row vector (2-D)
  Reshape1 : Reshape  OutputDimensionality=Row vector (2-D)
  Sum4 : Sum  Inputs=|+-
  Sum5 : Sum  Inputs=|+-
  Switch : Switch  Criteria=u2 > Threshold
  Switch1 : Switch  Criteria=u2 > Threshold
  Proj : Outport
  wires:
  Divide1/1 -> Product7/2
  [theta] -> Product7/1
  Product7/1 -> [df]
  Product6/1 -> Divide1/2
  Math Function1/1 -> Product6/2
  [Thetamax] -> Math Function1/1
  Gain/1 -> Divide1/1
  Bias1/1 -> Gain/1
  [epsilontheta] -> Product6/1, Bias1/1
  [epsilontheta] -> Bias/1
  Bias/1 -> Product3/1
  Product3/1 -> Sum4/1
  Divide/1 -> [f]
  Product2/1 -> Divide/2
  [epsilontheta] -> Product2/2
  epsilontheta/1 -> [epsilontheta]
  [Thetamax] -> Math Function/1
  Thetamax/1 -> [Thetamax]
  Dot Product/1 -> Product/2
  [y] -> Dot Product/2
  Normalize Vector1/1 -> Product/1, Dot Product/1
  [df] -> Normalize Vector1/1
  [f] -> Product1/2
  Sum5/1 -> Switch1/1
  Product1/1 -> Sum5/2
  [y] -> Switch1/3
  Product/1 -> Product1/1
  [y] -> Sum5/1
  Switch1/1 -> Switch/1
  [y] -> Switch/3
  theta/1 -> [theta]
  Reshape1/1 -> Product4/1
  Reshape/1 -> Product5/1
  [df] -> Reshape/1
  [theta] -> Product4/2, Reshape1/1
  Product4/1 -> Product3/2
  Math Function/1 -> Product2/1, Sum4/2
  Sum4/1 -> Divide/1
  [y] -> Product5/2
  Product5/1 -> Switch1/2
  Switch/1 -> Proj/1
  y/1 -> [y]
  [f] -> Switch/2
